simulink model "TP3_3_1_1"  (R2025b)
settings: Solver=VariableStepAuto  StartTime=0.0  StopTime=10.0  RelTol=1e-3
undefined symbols (not defined in the file): Bm_val, Jm_val, Kc_val, Km_val, L_val, R_val
settings Model: Creator=diegoalfonsocosta  LastModifiedBy=diegoalfonsocosta

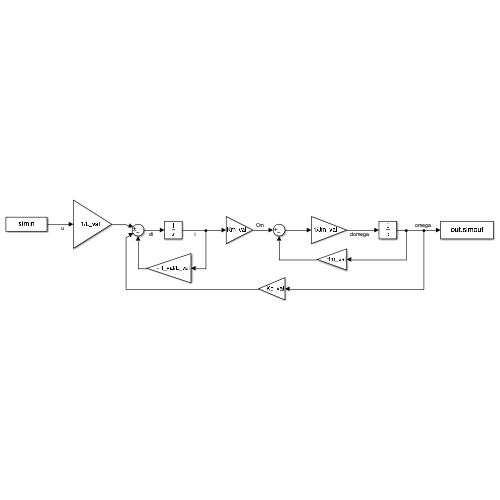
[thumbnail: Simulink's stored preview of the top-level diagram]
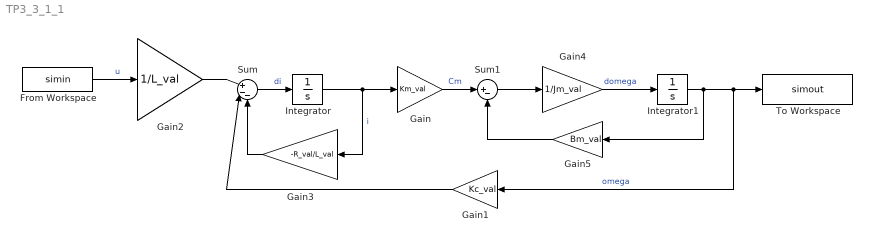
== system TP3_3_1_1 ==
  From Workspace : FromWorkspace  VariableName=simin
  Gain : Gain  Gain=Km_val
  Gain1 : Gain  Gain=Kc_val
  Gain2 : Gain  Gain=1/L_val
  Gain3 : Gain  Gain=-R_val/L_val
  Gain4 : Gain  Gain=1/Jm_val
  Gain5 : Gain  Gain=Bm_val
  Integrator : Integrator
  Integrator1 : Integrator
  Sum : Sum  Inputs=|+--
  Sum1 : Sum  Inputs=|+-
  To Workspace : ToWorkspace  VariableName=simout  SaveFormat=Timeseries  SampleTime=-1
  wires:
  Integrator/1 -> Gain3/1, Gain/1  "i"
  Gain/1 -> Sum1/1  "Cm"
  Integrator1/1 -> Gain5/1, To Workspace/1, Gain1/1  "omega"
  From Workspace/1 -> Gain2/1  "u"
  Sum/1 -> Integrator/1  "di"
  Gain2/1 -> Sum/1
  Gain1/1 -> Sum/2
  Gain3/1 -> Sum/3
  Sum1/1 -> Gain4/1
  Gain4/1 -> Integrator1/1  "domega"
  Gain5/1 -> Sum1/2
